simulink subsystem "Day6_Scenario_1"  (R2024a)
settings: Solver=VariableStepAuto  StartTime=0.0  StopTime=10.0  RelTol=1e-3
libraries: CarMaker4SL x10
settings Model: Creator=junhyung.cha  LastModifiedBy=junhyung.cha

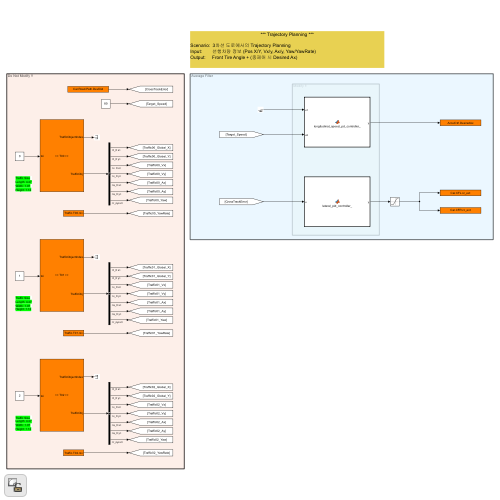
[thumbnail: Simulink's stored preview of the top-level diagram]
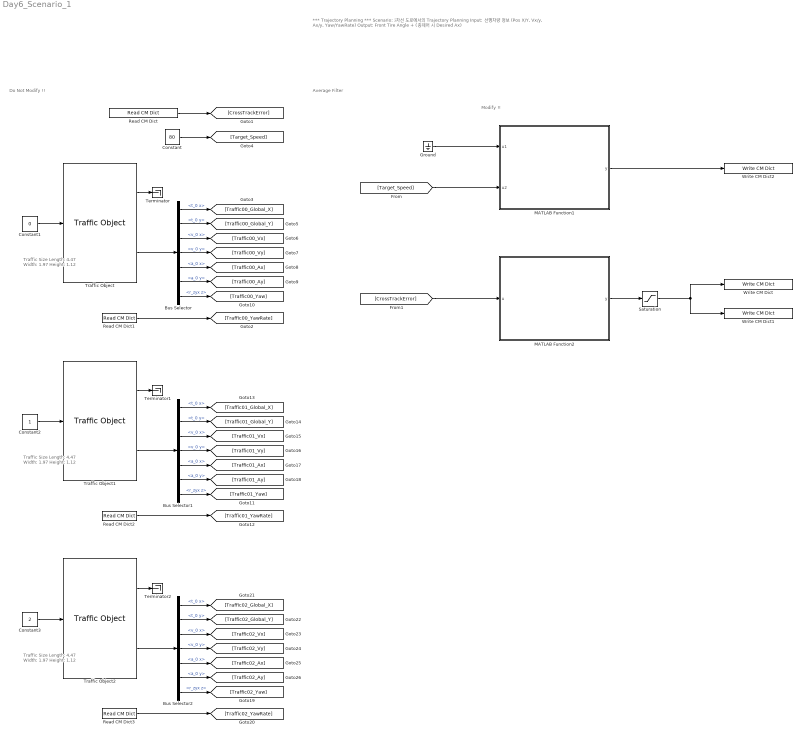
== system Day6_Scenario_1 ==
  note: Average Filter
  note: Do Not Modify !!
  note: Traffic Size
      | Length: 4.47
      | Width: 1.97
      | Height: 1.12
  note: Modify !!
  note: Traffic Size
      | Length: 4.47
      | Width: 1.97
      | Height: 1.12
  note: Traffic Size
      | Length: 4.47
      | Width: 1.97
      | Height: 1.12
  note: *** Trajectory Planning ***
      |
      | Scenario: 3차선 도로에서의 Trajectory Planning
      | Input: 선행차량 정보 (Pos X/Y, Vx/y, Ax/y, Yaw/YawRate)
      | Output: Front Tire Angle + (종제어 시 Desired Ax)
  Bus Selector : BusSelector  OutputSignals=t_0 x,t_0 y,v_0 x,v_0 y,a_0 x,a_0 y,r_zyx z
  Bus Selector1 : BusSelector  OutputSignals=t_0 x,t_0 y,v_0 x,v_0 y,a_0 x,a_0 y,r_zyx z
  Bus Selector2 : BusSelector  OutputSignals=t_0 x,t_0 y,v_0 x,v_0 y,a_0 x,a_0 y,r_zyx z
  Constant : Constant  Value=80
  Constant1 : Constant  Value=0
  Constant2 : Constant
  Constant3 : Constant  Value=2
  Ground : Ground
  MATLAB Function1 : MATLAB Function  TreatAsAtomicUnit=on
  MATLAB Function2 : MATLAB Function  TreatAsAtomicUnit=on
  Read CM Dict : CarMaker4SL/Read CM Dict  xname=Car.Road.Path.DevDist  xsync=off  xstime=Inherited
  Read CM Dict1 : CarMaker4SL/Read CM Dict  xname=Traffic.T00.rzv  xsync=off  xstime=Inherited
  Read CM Dict2 : CarMaker4SL/Read CM Dict  xname=Traffic.T01.rzv  xsync=off  xstime=Inherited
  Read CM Dict3 : CarMaker4SL/Read CM Dict  xname=Traffic.T02.rzv  xsync=off  xstime=Inherited
  Saturation : Saturate  UpperLimit=2  LowerLimit=-2
  Terminator : Terminator
  Terminator1 : Terminator
  Terminator2 : Terminator
  Traffic Object : CarMaker4SL/Traffic Object  xname=T00  ximode=Traffic Id  xstime=Inherited
      settings: SourceProductName=CarMaker4SL
  Traffic Object1 : CarMaker4SL/Traffic Object  xname=T01  ximode=Traffic Id  xstime=Inherited
      settings: SourceProductName=CarMaker4SL
  Traffic Object2 : CarMaker4SL/Traffic Object  xname=T02  ximode=Traffic Id  xstime=Inherited
      settings: SourceProductName=CarMaker4SL
  Write CM Dict : CarMaker4SL/Write CM Dict  xname=Car.CFL.rz_ext  xsync=off
  Write CM Dict1 : CarMaker4SL/Write CM Dict  xname=Car.CFR.rz_ext  xsync=off
  Write CM Dict2 : CarMaker4SL/Write CM Dict  xname=AccelCtrl.DesiredAx  xsync=off
  wires:
  Saturation/1 -> Write CM Dict1/1, Write CM Dict/1
  Constant1/1 -> Traffic Object/1
  MATLAB Function2/1(y) -> Saturation/1
  MATLAB Function1/1(y) -> Write CM Dict2/1
  [CrossTrackError] -> MATLAB Function2/1(u)
  Ground/1 -> MATLAB Function1/1(u1)
  Read CM Dict/1 -> [CrossTrackError]
  [Target_Speed] -> MATLAB Function1/2(u2)
  Constant/1 -> [Target_Speed]
  Bus Selector/4 -> [Traffic00_Vy]  "<v_0 y>"
  Traffic Object/1 -> Terminator/1
  Bus Selector/3 -> [Traffic00_Vx]  "<v_0 x>"
  Traffic Object/2 -> Bus Selector/1
  Bus Selector/1 -> [Traffic00_Global_X]  "<t_0 x>"
  Bus Selector/2 -> [Traffic00_Global_Y]  "<t_0 y>"
  Read CM Dict1/1 -> [Traffic00_YawRate]
  Bus Selector/5 -> [Traffic00_Ax]  "<a_0 x>"
  Bus Selector/6 -> [Traffic00_Ay]  "<a_0 y>"
  Bus Selector/7 -> [Traffic00_Yaw]  "<r_zyx z>"
  Read CM Dict2/1 -> [Traffic01_YawRate]
  Bus Selector1/1 -> [Traffic01_Global_X]  "<t_0 x>"
  Bus Selector1/5 -> [Traffic01_Ax]  "<a_0 x>"
  Bus Selector1/6 -> [Traffic01_Ay]  "<a_0 y>"
  Bus Selector1/7 -> [Traffic01_Yaw]  "<r_zyx z>"
  Traffic Object1/1 -> Terminator1/1
  Bus Selector1/4 -> [Traffic01_Vy]  "<v_0 y>"
  Constant2/1 -> Traffic Object1/1
  Traffic Object1/2 -> Bus Selector1/1
  Bus Selector1/3 -> [Traffic01_Vx]  "<v_0 x>"
  Bus Selector1/2 -> [Traffic01_Global_Y]  "<t_0 y>"
  Bus Selector2/3 -> [Traffic02_Vx]  "<v_0 x>"
  Bus Selector2/2 -> [Traffic02_Global_Y]  "<t_0 y>"
  Traffic Object2/2 -> Bus Selector2/1
  Bus Selector2/1 -> [Traffic02_Global_X]  "<t_0 x>"
  Bus Selector2/6 -> [Traffic02_Ay]  "<a_0 y>"
  Constant3/1 -> Traffic Object2/1
  Traffic Object2/1 -> Terminator2/1
  Bus Selector2/7 -> [Traffic02_Yaw]  "<r_zyx z>"
  Bus Selector2/5 -> [Traffic02_Ax]  "<a_0 x>"
  Read CM Dict3/1 -> [Traffic02_YawRate]
  Bus Selector2/4 -> [Traffic02_Vy]  "<v_0 y>"

== matlab function Day6_Scenario_1/MATLAB Function2 ==
  settings: sampleTime=0.1
  data: u input; y output
function y = lateral_pid_controller_(u)
    y = 0;
end

== matlab function Day6_Scenario_1/MATLAB Function1 ==
  settings: sampleTime=0.1
  data: u1 input; y output; u2 input
function y = longitudinal_speed_pd_controller_(u1, u2)
    y = 0;
end
